simulink model "Delay_Discrete"  (Simulink 8.0)
settings: Solver=ode45  StartTime=0.0  StopTime=10.0  RelTol=1e-3
libraries: simulink x2
settings Model: Creator=Faradars  LastModifiedBy=Faradars

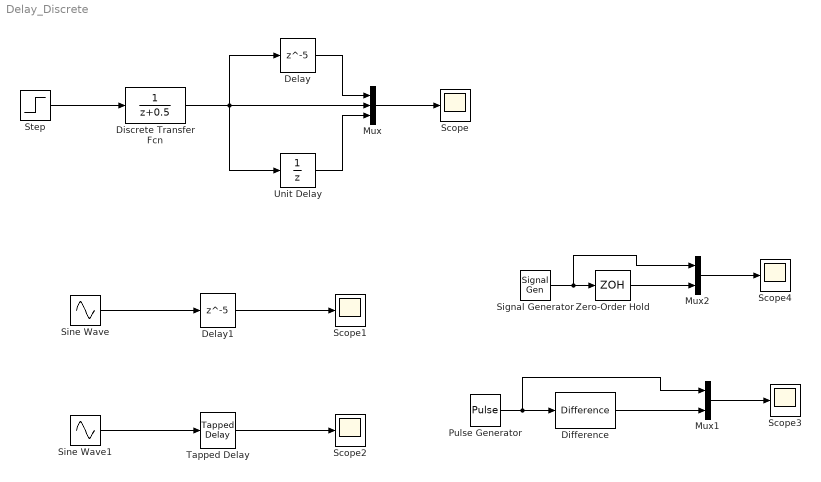
== system Delay_Discrete ==
  Delay : Delay  DelayLength=5  SampleTime=0.3
  Delay1 : Delay  DelayLength=5  SampleTime=0.1
  Difference : simulink/Discrete/Difference  ICPrevInput=0.05  InputProcessing=Inherited  OutMin=[]  OutMax=[]  OutDataType=fixdt(1, 16)  OutScaling=2^-10  DoSatur=off
  Discrete Transfer Fcn : DiscreteTransferFcn  SampleTime=0.2
  Mux : Mux  Inputs=3
  Mux1 : Mux  Inputs=2
  Mux2 : Mux  Inputs=2
  Pulse Generator : DiscretePulseGenerator  PulseType=Time based  Period=4  PulseWidth=50
  Scope{,1..4} (5 alike) : Scope
      Scope2 settings: SaveName=ScopeData2
      Scope3 settings: SaveName=ScopeData3
      Scope4 settings: SaveName=ScopeData4
  Signal Generator : SignalGenerator  WaveForm=random
  Sine Wave : Sin  SampleTime=0.1
  Sine Wave1 : Sin  SampleTime=0.1
  Step : Step  SampleTime=0.2
  Tapped Delay : simulink/Discrete/Tapped Delay  vinit=0.0  samptime=0.1  NumDelays=4  DelayOrder=Oldest  includeCurrent=off
  Unit Delay : UnitDelay  SampleTime=0.5
  Zero-Order Hold : ZeroOrderHold  SampleTime=0.5
  wires:
  Discrete Transfer Fcn/1 -> Delay/1, Unit Delay/1, Mux/2
  Step/1 -> Discrete Transfer Fcn/1
  Mux/1 -> Scope/1
  Delay/1 -> Mux/1
  Unit Delay/1 -> Mux/3
  Sine Wave/1 -> Delay1/1
  Delay1/1 -> Scope1/1
  Sine Wave1/1 -> Tapped Delay/1
  Tapped Delay/1 -> Scope2/1
  Pulse Generator/1 -> Mux1/1, Difference/1
  Difference/1 -> Mux1/2
  Mux1/1 -> Scope3/1
  Signal Generator/1 -> Mux2/1, Zero-Order Hold/1
  Mux2/1 -> Scope4/1
  Zero-Order Hold/1 -> Mux2/2
